simulink model "modelSStemp"  (R2021b)
settings: Solver=VariableStepAuto  StartTime=0.0  StopTime=10.0  RelTol=1e-3
undefined symbols (not defined in the file or in its folder): A, B, B_d, C, K, T_AMBIENT
settings Model: Creator=martin  LastModifiedBy=martin

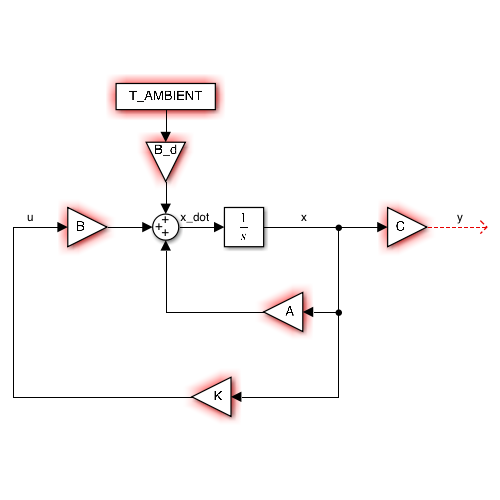
[thumbnail: Simulink's stored preview of the top-level diagram]
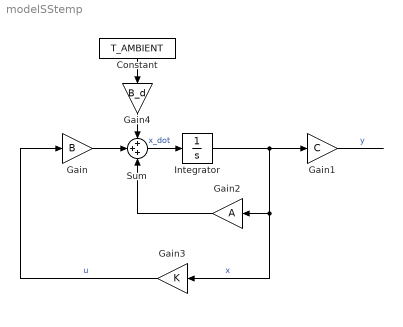
== system modelSStemp ==
  Constant : Constant  Value=T_AMBIENT
  Gain : Gain  Gain=B
  Gain1 : Gain  Gain=C
  Gain2 : Gain  Gain=A
  Gain3 : Gain  Gain=K
  Gain4 : Gain  Gain=B_d
  Integrator : Integrator
  Sum : Sum  Inputs=+++
  wires:
  Sum/1 -> Integrator/1  "x_dot"
  Integrator/1 -> Gain3/1, Gain2/1, Gain1/1  "x"
  Gain2/1 -> Sum/3
  Gain/1 -> Sum/2
  Gain3/1 -> Gain/1  "u"
  Gain1/1 -> ?  "y"
  Constant/1 -> Gain4/1
  Gain4/1 -> Sum/1
